simulink model "simu_final"  (R2018b)
settings: Solver=FixedStepAuto  StartTime=0.0  StopTime=0.5  FixedStep=0.001  RelTol=1e-3
values from neighbouring files (symbols this model uses):
  C = tf([ (Kp + Kd*f) Kp*f ],[1 f])    [calculos.m]
  D = tf([wn^2],[1 2*zeta*wn wn^2])    [calculos.m]
  G = tf([ c3 ],[ 1 c4 0 ])    [calculos.m]
settings Model: Creator=lubuntu  LastModifiedBy=lubuntu

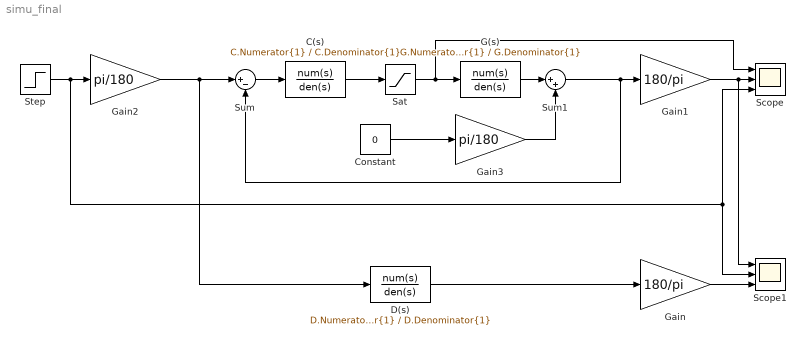
== system simu_final ==
  C(s) : TransferFcn  Numerator=C.Numerator{1}  Denominator=C.Denominator{1}
  Constant : Constant  Value=0
  D(s) : TransferFcn  Numerator=D.Numerator{1}  Denominator=D.Denominator{1}
  G(s) : TransferFcn  Numerator=G.Numerator{1}  Denominator=G.Denominator{1}
  Gain : Gain  Gain=180/pi
  Gain1 : Gain  Gain=180/pi
  Gain2 : Gain  Gain=pi/180
  Gain3 : Gain  Gain=pi/180
  Sat : Saturate  UpperLimit=7  LowerLimit=-7
  Scope : Scope  NumInputPorts=3
  Scope1 : Scope  NumInputPorts=3
  Step : Step  Time=0.001  Before=-10  After=10  SampleTime=0
  Sum : Sum  Inputs=|+-
  Sum1 : Sum  Inputs=|++
  wires:
  Sum/1 -> C(s)/1
  C(s)/1 -> Sat/1
  Step/1 -> Scope/3, Scope1/2, Gain2/1
  D(s)/1 -> Gain/1
  Sat/1 -> Scope/1, G(s)/1
  Gain1/1 -> Scope1/1, Scope/2
  Gain/1 -> Scope1/3
  Gain2/1 -> D(s)/1, Sum/1
  G(s)/1 -> Sum1/1
  Sum1/1 -> Sum/2, Gain1/1
  Constant/1 -> Gain3/1
  Gain3/1 -> Sum1/2
